simulink model "hw9c"  (R2021b)
settings: Solver=VariableStepAuto  StartTime=0.0  StopTime=50  MaxStep=0.001  RelTol=1e-3
settings Model: Creator=user  LastModifiedBy=user

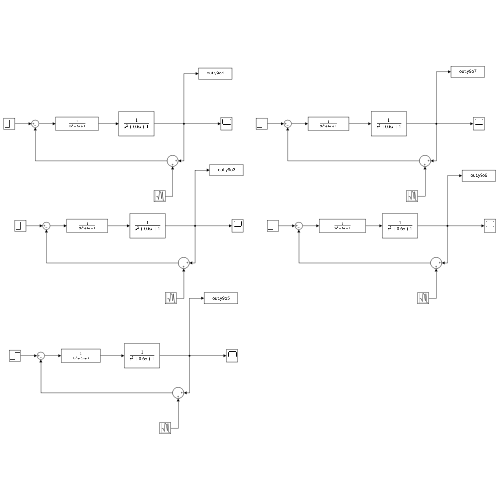
[thumbnail: Simulink's stored preview of the top-level diagram]
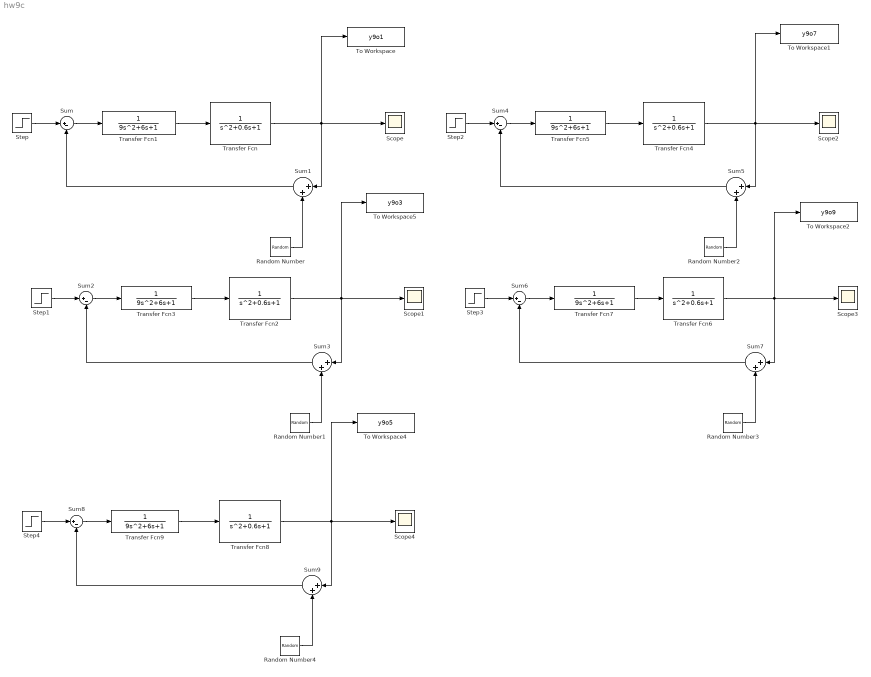
== system hw9c ==
  Random Number : RandomNumber  Variance=0.1  SampleTime=0.001
  Random Number1 : RandomNumber  Variance=0.3  SampleTime=0.001
  Random Number2 : RandomNumber  Variance=0.7  SampleTime=0.001
  Random Number3 : RandomNumber  Variance=0.9  SampleTime=0.001
  Random Number4 : RandomNumber  Variance=0.5  SampleTime=0.001
  Scope{,1..4} (5 alike) : Scope
  Step{,1..4} (5 alike) : Step  Time=0  SampleTime=0
  Sum{,2,4,6,8} (5 alike) : Sum  Inputs=|+-
  Sum{1,3,5,7,9} (5 alike) : Sum  Inputs=|++
  To Workspace : ToWorkspace  VariableName=y9o1  SaveFormat=Timeseries  SampleTime=-1
  To Workspace1 : ToWorkspace  VariableName=y9o7  SaveFormat=Timeseries  SampleTime=-1
  To Workspace2 : ToWorkspace  VariableName=y9o9  SaveFormat=Timeseries  SampleTime=-1
  To Workspace4 : ToWorkspace  VariableName=y9o5  SaveFormat=Timeseries  SampleTime=-1
  To Workspace5 : ToWorkspace  VariableName=y9o3  SaveFormat=Timeseries  SampleTime=-1
  Transfer Fcn{,2,4,6,8} (5 alike) : TransferFcn  Denominator="[1  0.6 1]"
  Transfer Fcn{1,3,5,7,9} (5 alike) : TransferFcn  Denominator=[9 6 1]
  wires:
  Sum2/1 -> Transfer Fcn3/1
  Transfer Fcn2/1 -> To Workspace5/1, Scope1/1, Sum3/1
  Step2/1 -> Sum4/1
  Transfer Fcn8/1 -> To Workspace4/1, Scope4/1, Sum9/1
  Step/1 -> Sum/1
  Transfer Fcn7/1 -> Transfer Fcn6/1
  Step4/1 -> Sum8/1
  Random Number2/1 -> Sum5/2
  Step3/1 -> Sum6/1
  Sum9/1 -> Sum8/2
  Transfer Fcn1/1 -> Transfer Fcn/1
  Transfer Fcn9/1 -> Transfer Fcn8/1
  Sum8/1 -> Transfer Fcn9/1
  Random Number3/1 -> Sum7/2
  Transfer Fcn/1 -> To Workspace/1, Scope/1, Sum1/1
  Transfer Fcn4/1 -> To Workspace1/1, Scope2/1, Sum5/1
  Random Number4/1 -> Sum9/2
  Sum6/1 -> Transfer Fcn7/1
  Sum5/1 -> Sum4/2
  Transfer Fcn6/1 -> To Workspace2/1, Scope3/1, Sum7/1
  Transfer Fcn5/1 -> Transfer Fcn4/1
  Step1/1 -> Sum2/1
  Sum/1 -> Transfer Fcn1/1
  Random Number1/1 -> Sum3/2
  Sum4/1 -> Transfer Fcn5/1
  Transfer Fcn3/1 -> Transfer Fcn2/1
  Sum3/1 -> Sum2/2
  Sum7/1 -> Sum6/2
  Random Number/1 -> Sum1/2
  Sum1/1 -> Sum/2
